simulink subsystem "multirotor_dynamic_model_sim"  (R2023b)
settings: Solver=VariableStepAuto  StartTime=0.0  StopTime=10.0  RelTol=1e-3
settings Model: Creator=minu_  LastModifiedBy=yizho

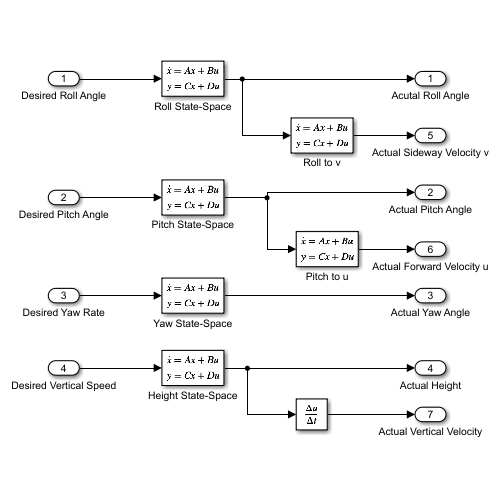
[thumbnail: Simulink's stored preview of the top-level diagram]
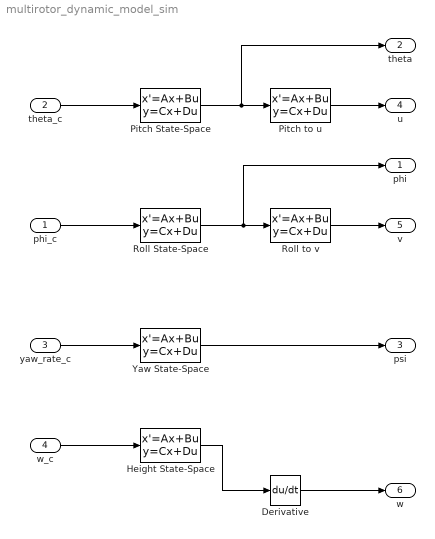
== system multirotor_dynamic_model_sim ==
  phi_c : Inport
  theta_c : Inport  Port=2
  yaw_rate_c : Inport  Port=3
  w_c : Inport  Port=4
  Derivative : Derivative
  Height State-Space : StateSpace  A=[-5.8200 -3.6046e-6; 3.8147e-6 0]  B=[1024; 0]  C=[1.4907e-4 1.3191e3]  D=0  InitialCondition=0
  Pitch State-Space : StateSpace  A=[-3.9784, -2.9796; 4, 0]  B=[2; 0]  C=[1.2569, 0.6083]  D=0  InitialCondition=0
  Pitch to u : StateSpace  A=[-0.665]  B=[2]  C=[-3.0772]  D=0  InitialCondition=0
  Roll State-Space : StateSpace  A=[-4.2683 -3.1716; 4 0]  B=[2; 0]  C=[0.7417 0.4405]  D=0  InitialCondition=0
  Roll to v : StateSpace  A=[-0.4596]  B=[2]  C=[2.3868]  D=0  InitialCondition=0
  Yaw State-Space : StateSpace  A=[-0.0059]  B=[1]  C=[1.2653]  D=0  InitialCondition=0
  phi : Outport
  theta : Outport  Port=2
  psi : Outport  Port=3
  u : Outport  Port=4
  v : Outport  Port=5
  w : Outport  Port=6
  wires:
  Pitch State-Space/1 -> Pitch to u/1, theta/1
  Derivative/1 -> w/1
  Roll State-Space/1 -> Roll to v/1, phi/1
  theta_c/1 -> Pitch State-Space/1
  w_c/1 -> Height State-Space/1
  yaw_rate_c/1 -> Yaw State-Space/1
  phi_c/1 -> Roll State-Space/1
  Height State-Space/1 -> Derivative/1
  Pitch to u/1 -> u/1
  Roll to v/1 -> v/1
  Yaw State-Space/1 -> psi/1
